simulink model "sm_humanoid_walker_ga"  (R2022b)
settings: Solver=daessc  StartTime=0.0  StopTime=params.simulation.Tf  RelTol=1e-3  AbsTol=1e-3
model workspace (MATLAB code in the model file):
  | sm_humanoid_walker_ga_parameters;
  | 
  | if ~exist('x','var')
  |       x = [0.9182    0.9441    0.6705   -0.2348   -0.2725   ...
  |         -1.0000   -0.9120    0.5830   -0.1476    0.5914   ...
  |         -0.5010   -0.7179    1.3537];
  |     nPoints = 4;
  |     %Process solution
  |     waypoints = sm_humanoid_walker_generate_waypoints(x(1:end-1),nPoints);
  |     gaitPeriod = x(end);
  |     clear x nPoints
  | end
undefined symbols (not defined in the file or in its folder): params, X, Y, Z
libraries: sm_humanoid_walker_lib x5, sm_lib x4, simulink x1, nesl_utility x1
settings Model: Creator=The MathWorks, Inc.  LastModifiedBy=The MathWorks, Inc.
settings SolverCC: AlgebraicLoopSolver=TrustRegion
settings DebuggingCC: ParameterPrecisionLossMsg=none  ParameterTunabilityLossMsg=none  UnconnectedInputMsg=warning  UnconnectedOutputMsg=warning  UnconnectedLineMsg=warning  SFMachineParentedDataDiag=warning
settings ModelReferenceCC: EnableRefExpFcnMdlSchedulingChecks=on
settings RTWCC: DLArmComputeVersion=19.05
settings ExplorerConfigSet: InternalSimMechanicsExplorerSettings="<ExplorerConfiguration><canonicalview>default</canonicalview><AnimationSetting><BasePlaybackSpeed>1.0</BasePlaybackSpeed><PlaybackSpeedFactor>1.0</PlaybackSpeedFactor></AnimationSetting><TilePanel><TileInfo><Tiles Columns=\"1\" Count=\"1\" Rows=\"1\"><Column Weight=\"1\"/><Row Weight=\"1\"/><Tile Height=\"1\" Width=\"1\" X=\"0\" Y=\"0\"/></Tiles></TileInfo><SceneInfo><SceneViewer><BGColor><R>0.800000011920928955</R><G>1</G><B>1</B></BGColor><Camera><DoPerspective>off</DoPerspective><Position><X>9.33069970005120908</X><Y>-28.3771970803646205</Y><Z>5.78557240639865533</Z></Position><Center><X>-5.66642883683167398</X><Y>-8.1624733210025866</Y><Z>-0.0320163947652276626</Z></Center><Up><X>-0.138282834726365628</X><Y>0.177803146917367316</Y><Z>0.974301749237022729</Z></Up><ViewLimDist>1</ViewLimDist><YLim>3.97770924405576354</YLim><XLim>6.09227752938848699</XLim></Camera></SceneViewer></SceneInfo></TilePanel><MechEditorPanel><Cameras><Camera><Id>Camera1</Id><Value><Name>Follow Cam</Name><NativeCamera><PositionKeyframeSet><Keyframe><Time>0</Time><Value><X>5.2204627070338789</X><Y>-24.273411935987699</Y><Z>0.88759148871818205</Z></Value></Keyframe><Keyframe><Time>3.2652976270560012</Time><Value><X>5.3496192797707485</X><Y>-21.54780848897293</Y><Z>0.90561457614580099</Z></Value></Keyframe><Keyframe><Time>11.604918208612045</Time><Value><X>6.8873790757613955</X><Y>-4.6901780376259916</Y><Z>1.7435854496631411</Z></Value></Keyframe><Keyframe><Time>20.826445213600746</Time><Value><X>0.0055188610359192848</X><Y>8.7825410723727551</Y><Z>3.6394031449856099</Z></Value></Keyframe><Keyframe><Time>27.488802341030855</Time><Value><X>-0.11347989269831198</X><Y>8.3449030154483967</Y><Z>9.2323195248135992</Z></Value></Keyframe><Keyframe><Time>32.87337148588913</Time><Value><X>-5.5799174331031223</X><Y>7.4045167178687716</Y><Z>2.0521136721648428</Z></Value></Keyframe><Keyframe><Time>41.966030622938355</Time><Value><X>-4.2975164122566225</X><Y>19.602249329555761</Y><Z>1.7418928889156724</Z></Value></Keyframe></PositionKeyframeSet><CenterKeyframeSet><Keyframe><Time>0</Time><Value><X>0.94511897384819221</X><Y>-24.070468135395043</Y><Z>0.83457179388827374</Z></Value></Keyframe><Keyframe><Time>3.2652976270560012</Time><Value><X>1.0742755465850635</X><Y>-21.34486468838028</Y><Z>0.85259488131589301</Z></Value></Keyframe><Keyframe><Time>11.604918208612045</Time><Value><X>-0.53078491432740638</X><Y>-10.107899469288508</Y><Z>0.98015389679796794</Z></Value></Keyframe><Keyframe><Time>20.826445213600746</Time><Value><X>-0.0093883253568207564</X><Y>-0.37419006503563246</Y><Z>1.1555147927727409</Z></Value></Keyframe><Keyframe><Time>27.488802341030855</Time><Value><X>-0.16176080895536168</X><Y>7.8320516127470299</Y><Z>0.032557410765059913</Z></Value></Keyframe><Keyframe><Time>32.87337148588913</Time><Value><X>0.65386303236123666</X><Y>12.717291953789552</Y><Z>0.85437963274956452</Z></Value></Keyframe><Keyframe><Time>41.966030622938355</Time><Value><X>-1.3921216836808661</X><Y>22.07838868833927</Y><Z>1.1836617828265599</Z></Value></Keyframe></CenterKeyframeSet><UpVectorKeyframeSet><Keyframe><Time>0</Time><Value><X>-0.012685369434117804</X><Y>-0.0060107470198237194</Y><Z>0.99990147130734031</Z></Value></Keyframe><Keyframe><Time>3.2652976270560012</Time><Value><X>-0.012685369434116568</X><Y>-0.0060107470198237783</Y><Z>0.99990147130734042</Z></Value></Keyframe><Keyframe><Time>11.604918208612045</Time><Value><X>-0.0869845609404266</X><Y>-0.021244943951286073</Y><Z>0.99598310152055713</Z></Value></Keyframe><Keyframe><Time>20.826445213600746</Time><Value><X>-0.0025118121577261984</X><Y>-0.26179775052186577</Y><Z>0.96511948929724511</Z></Value></Keyframe><Keyframe><Time>27.488802341030855</Time><Value><X>-0.0021877954754526627</X><Y>-0.9984467673798999</Y><Z>0.055671054054916028</Z></Value></Keyframe><Keyframe><Time>32.87337148588913</Time><Value><X>0.14201921265768605</X><Y>0.056160365220433037</Y><Z>0.98826947570710622</Z></Value></Keyframe><Keyframe><Time>41.966030622938355</Time><Value><X>0.14201921265768569</X><Y>0.056160365220432724</Y><Z>0.98826947570710644</Z></Value></Keyframe></UpVectorKeyframeSet></NativeCamera></Value></Camera></Cameras><GfxPanelCameraMap/><VideoCreator><PlaybackSpeedRatio>1.0</PlaybackSpeedRatio><FrameRate>30</FrameRate><VideoFormat>Motion JPEG AVI</VideoFormat><FrameSize>auto</FrameSize></VideoCreator></MechEditorPanel></ExplorerConfiguration>"

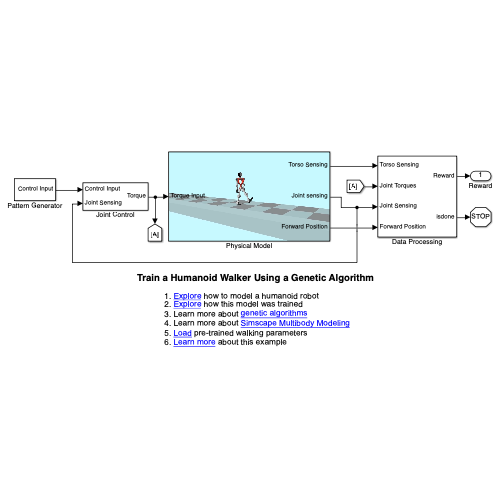
[thumbnail: Simulink's stored preview of the top-level diagram]
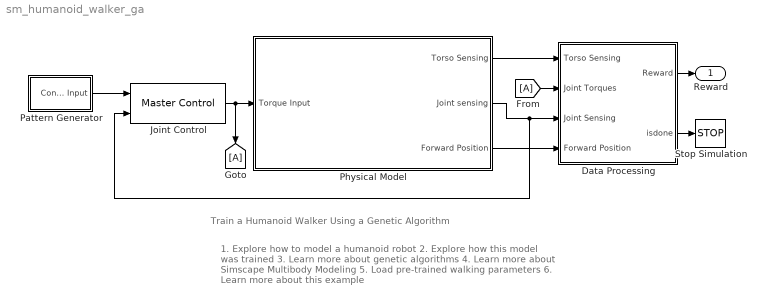
== system sm_humanoid_walker_ga ==
  note: Train a Humanoid Walker Using a Genetic Algorithm
  note: 1. Explore how to model a humanoid robot
      | 2. Explore how this model was trained
      | 3. Learn more about genetic algorithms
      | 4. Learn more about Simscape Multibody Modeling
      | 5. Load pre-trained walking parameters
      | 6. Learn more about this example
  Data Processing : Subsystem
  From : From
  Goto : Goto
  Joint Control : sm_humanoid_walker_lib/Master Control  SystemSampleTime=-1  VariantActivationTime=update diagram  Latency=0  AutoFrameSizeCalculation=off
  Pattern Generator : Subsystem
  Physical Model : Subsystem
      mask Display: image('imagebackground.PNG'); % Use "Edit Image" on toolstrip to change.
  Stop Simulation : Stop
  Reward : Outport
  wires:
  Data Processing/1(Reward) -> Reward/1
  Physical Model/1(Torso Sensing) -> Data Processing/1(Torso Sensing)
  Pattern Generator/1(Control Input) -> Joint Control/1
  Physical Model/2(Joint sensing) -> Joint Control/2, Data Processing/3(Joint Sensing)
  Data Processing/2(isdone) -> Stop Simulation/1
  Physical Model/3(Forward Position) -> Data Processing/4(Forward Position)
  Joint Control/1 -> Physical Model/1(Torque Input), Goto/1
  From/1 -> Data Processing/2(Joint Torques)

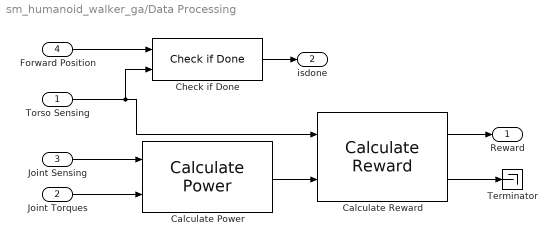
== system sm_humanoid_walker_ga/Data Processing ==
  Torso Sensing : Inport
  Joint Torques : Inport  Port=2
  Joint Sensing : Inport  Port=3
  Forward Position : Inport  Port=4
  Calculate Power : sm_humanoid_walker_lib/Calculate Power  SystemSampleTime=-1  VariantActivationTime=update diagram  Latency=0  AutoFrameSizeCalculation=off
  Calculate Reward : sm_humanoid_walker_lib/Calculate Reward  forwardReward=params.reward.forwardRewardWeight  timestepReward=params.reward.timestepRewardWeight  powerPenalty=params.reward.powerPenaltyWeight  verticalPenalty=params.reward.verticalPenaltyWeight  lateralPenalty=params.reward.lateralPenaltyWeight
  Check if Done : sm_humanoid_walker_lib/Check if Done  verticalStop=params.stoppingCriteria.heightChange  lateralStop=params.stoppingCriteria.lateral  angularStop=params.stoppingCriteria.angle  timeoutTime=params.stoppingCriteria.timeoutTime  timeoutDistance=params.stoppingCriteria.timeoutDistance
  Terminator : Terminator
  Reward : Outport
  isdone : Outport  Port=2
  wires:
  Torso Sensing/1 -> Check if Done/2, Calculate Reward/1
  Check if Done/1 -> isdone/1
  Calculate Power/1 -> Calculate Reward/2
  Joint Sensing/1 -> Calculate Power/1
  Joint Torques/1 -> Calculate Power/2
  Calculate Reward/1 -> Reward/1
  Forward Position/1 -> Check if Done/1
  Calculate Reward/2 -> Terminator/1

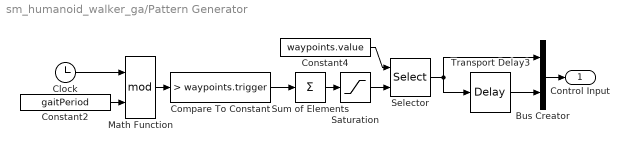
== system sm_humanoid_walker_ga/Pattern Generator ==
  Bus Creator : BusCreator  Inputs=2
  Clock : Clock
  Compare To Constant : simulink/Logic and Bit Operations/Compare To Constant  relop=>  const=waypoints.trigger  OutDataTypeStr=boolean
  Constant2 : Constant  Value=gaitPeriod
  Constant4 : Constant  Value=waypoints.value
  Math Function : Math  Operator=mod
  Saturation : Saturate  UpperLimit=100  LowerLimit=1  ZeroCross=off
  Selector : Selector  NumberOfDimensions=2  InputPortWidth=3  IndexOptions=Select all,Index vector (port)  Indices=[1 3],1  OutputSizes=1,1
  Sum of Elements : Sum  Inputs=+
  Transport Delay3 : TransportDelay  DelayTime=gaitPeriod/2  BufferSize=4096
  Control Input : Outport
  wires:
  Transport Delay3/1 -> Bus Creator/2
  Bus Creator/1 -> Control Input/1
  Selector/1 -> Transport Delay3/1, Bus Creator/1
  Clock/1 -> Math Function/1
  Constant2/1 -> Math Function/2
  Math Function/1 -> Compare To Constant/1
  Compare To Constant/1 -> Sum of Elements/1
  Constant4/1 -> Selector/1
  Sum of Elements/1 -> Saturation/1
  Saturation/1 -> Selector/2

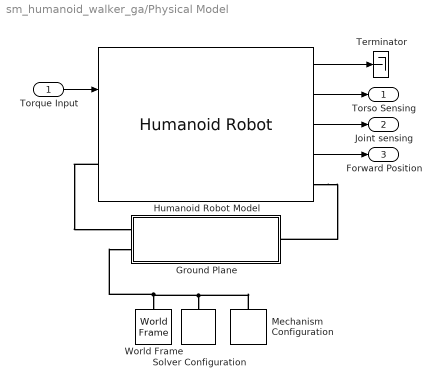
== system sm_humanoid_walker_ga/Physical Model ==
  Torque Input : Inport
  Ground Plane : Subsystem
  Humanoid Robot Model : sm_humanoid_walker_lib/Humanoid Robot  contactRadius=params.contact.contactRadius  contactStiffness=params.contact.stiffness  contactDamping=params.contact.damping  contactTWidth=params.contact.transitionWidth  contactStaticFriction=params.contact.staticFriction  contactDynamicFriction=params.contact.dynamicFriction  contactCriticalVelocity=params.contact.criticalVelocity  footDensity=params.materialProperties.lowerBodyDensity  lowerLegDensity=params.materialProperties.lowerBodyDensity  upperLegDensity=params.materialProperties.lowerBodyDensity  hipDensity=params.materialProperties.lowerBodyDensity  trunkDensity=params.materialProperties.upperBodyDensity  shoulderDensity=params.materialProperties.upperBodyDensity  upperArmDensity=params.materialProperties.upperBodyDensity  lowerArmDensity=params.materialProperties.upperBodyDensity  handDensity=params.materialProperties.upperBodyDensity  headDensity=params.materialProperties.upperBodyDensity  hipUpperLimit=params.jointLimits.hipFrontalUpperLimit  hipLowerLimit=params.jointLimits.hipFrontalLowerLimit  kneeUpperLimit=params.jointLimits.kneeUpperLimit  kneeLowerLimit=params.jointLimits.kneeLowerLimit  ankleUpperLimit=params.jointLimits.ankleUpperLimit  ankleLowerLimit=params.jointLimits.ankleLowerLimit  shoulderFrontalUpperLimit=params.jointLimits.shoulderFrontalUpperLimit  shoulderFrontalLowerLimit=params.jointLimits.shoulderFrontalLowerLimit  shoulderSagittalUpperLimit=params.jointLimits.shoulderSagittalUpperLimit  shoulderSagittalLowerLimit=params.jointLimits.shoulderSagittalLowerLimit
  Mechanism Configuration : sm_lib/Utilities/Mechanism Configuration  UniformGravity=Constant  GravityVector=[0 0 -9.80665]  GravityUnits=m/s^2  LinearizationDelta=0.001  JointModeTransitionNonlinearIterations=2
  Solver Configuration : nesl_utility/Solver Configuration  PhysicalDomain=network_engine_domain  SubClassName=solver  LeftPortType=input  RightPortType=generic  Tones=[]  Harmonics=[]  SimulateNoise=off  Profile=off  UseLocalSampling=off  EnableSwitchedLinearOptims=on  FrequencyDomain=off  UseCCode=off  RelTol=0.001  AbsTol=1e-06  MinStep=1e-09  ToWorkspace=off  RevertToSquareIcSolve=off  NumHomotopyIterations=100  PhasorMode=off  PhasorModeNumHarmonics=1  ConsistencySolver=NEWTON_FTOL  IndexReductionMethod=DerivativeReplacement  DoDC=off  ResidualTolerance=1e-09  ConsistencyTolSource=GLOBAL  ConsistencyAbsTol=0.001  ConsistencyRelTol=0.001  ConsistencyTolFactor=0.001  UseLocalSolver=off  LocalSolverChoice=NE_BACKWARD_EULER_ADVANCER  ResolveIndetEquations=on  FunctionEvalNumThread=1  LocalSolverSampleTime=0.001  DoFixedCost=off  MaxNonlinIter=3  MaxModeIter=2  ComputeImpulses=off  ImpulseIterations=2  LinearAlgebra=auto  LinearAlgebraNumThread=0  EquationFormulation=NE_TIME_EF  DelaysMemoryBudget=1024  AutomaticFiltering=on  FilteringTimeConstant=0.001  PartitionStorageMethod=AS_NEEDED  PartitionMemoryBudget=1024  PartitionMethod=ROBUST
  Terminator : Terminator
  World Frame : sm_lib/Frames and Transforms/World Frame
  Torso Sensing : Outport
  Joint sensing : Outport  Port=2
  Forward Position : Outport  Port=3
  wires:
  Humanoid Robot Model/2 -> Torso Sensing/1
  Humanoid Robot Model/1 -> Terminator/1
  Torque Input/1 -> Humanoid Robot Model/1
  Humanoid Robot Model/3 -> Joint sensing/1
  Humanoid Robot Model/4 -> Forward Position/1
  connections:
  Humanoid Robot Model/RConn1 -- Ground Plane/RConn1
  Mechanism Configuration/RConn1 -- World Frame/RConn1 -- Ground Plane/LConn2 -- Solver Configuration/RConn1
  Humanoid Robot Model/LConn1 -- Ground Plane/LConn1

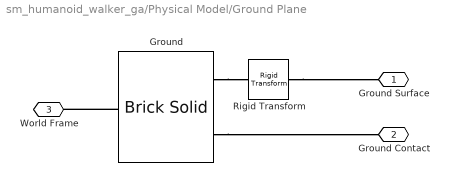
== system sm_humanoid_walker_ga/Physical Model/Ground Plane ==
  Ground : sm_lib/Body Elements/Brick Solid  GraphicAmbientColor=[0.15 0.15 0.15 1.0]  BasedOnType=Density  BrickDimensions=[params.display.planeWidth params.display.planeLength params.display.planeHeight]  BrickDimensionUnits=m  CenterOfMass=[0 0 0]  CenterOfMassUnits=m  GraphicDiffuseColor=params.display.floorColour  Density=1000  DensityUnits=kg/m^3  DoExposeReferenceFrame=on  GraphicEmissiveColor=[0.0 0.0 0.0 1.0]  ExportEntireGeometry=on  SerializedFrames=<Frames><Frame><Id>Frame1</Id><Value><Name>GS</Name><Origin><Source>GeometricFeature</Source><FeatureName>+z surface</FeatureName></Origin><PrimaryAxis><DefinedDirection>+Z</DefinedDirection><Source>ReferenceFrame</Source><SourceDirection>+Z</SourceDirection><FeatureName></FeatureName></PrimaryAxis><SecondaryAxis><DefinedDirection>+X</DefinedDirection><Source>ReferenceFrame</Source><SourceDirection>+X</SourceDirection><FeatureName></FeatureName></SecondaryAxis></Value></Frame></Frames>  MarkerShape=Sphere  MarkerSize=10  GraphicType=FromGeometry  InertiaType=CalculateFromGeometry  Mass=1  MassUnits=kg  MomentsOfInertia=[1 1 1]  MomentsOfInertiaUnits=kg*m^2  GraphicOpacity=0.3  ProductsOfInertia=[0 0 0]  ProductsOfInertiaUnits=kg*m^2  GraphicShininess=75  GraphicSpecularColor=[0.5 0.5 0.5 1.0]  GraphicVisPropType=SimpleVisualProperties
  Rigid Transform : sm_lib/Frames and Transforms/Rigid Transform  TranslationMethod=StandardAxis  TranslationStandardOffset=0.5-(params.display.planeLength/2)  TranslationLengthUnit=m  TranslationStandardAxis=+Y  TranslationCartesianOffset=[0 0 0]  TranslationROffset=0  TranslationROffsetUnits=m  TranslationZOffset=0  TranslationZOffsetUnits=m  TranslationThetaOffset=0  TranslationThetaOffsetUnits=deg  RotationMethod=None  RotationAngleUnits=deg  RotationStandardAxis=+Z  RotationAngle=0.0  RotationArbitraryAxis=[0 0 1]  FollAlignAxisA=+X  BaseAlignAxisA=+Y  FollAlignAxisB=+Y  BaseAlignAxisB=+Z  RotationSequenceAxes=FollowerAxes  RotationSequence=XYX  RotationSequenceAngles=[0 0 0]  RotationSequenceAnglesUnits=deg  RotationMatrix=[1 0 0; 0 1 0; 0 0 1]  Quaternion=[1 0 0 0]
  Ground Surface : PMIOPort  Side=Left
  Ground Contact : PMIOPort  Port=2  Side=Right
  World Frame : PMIOPort  Port=3  Side=Left
  connections:
  Ground/LConn1 -- Rigid Transform/LConn1
  Ground/LConn2 -- Ground Contact/RConn1
  Ground/RConn1 -- World Frame/RConn1
  Rigid Transform/RConn1 -- Ground Surface/RConn1
